simulink model "Appl_HeatAdj_CtrlModel"  (R2018b)
settings: configuration reference "CodeConfig_10_ms" (kept outside this file)
undefined symbols (not defined in the file): CAL_LEVEL3_TIMEOUT, CAL_SW_20min_TIMEOUT, D_1stLevel_36, D_2ndLevel_39, D_3rdLevel_45, D_3rdLevel_48, D_DRVHEAT_PID_D, D_DRVHEAT_PID_I, D_DRVHEAT_PID_P, D_HEAT_HEAT_DEF, D_SwsLevel_Temp, FALSE, TRUE
libraries: DareLib x111, simulink x1
(part 1 of 6)
settings Model: Creator=Administrator  LastModifiedBy=Administrator
settings ConfigSetRef: SourceLocation=Base Workspace

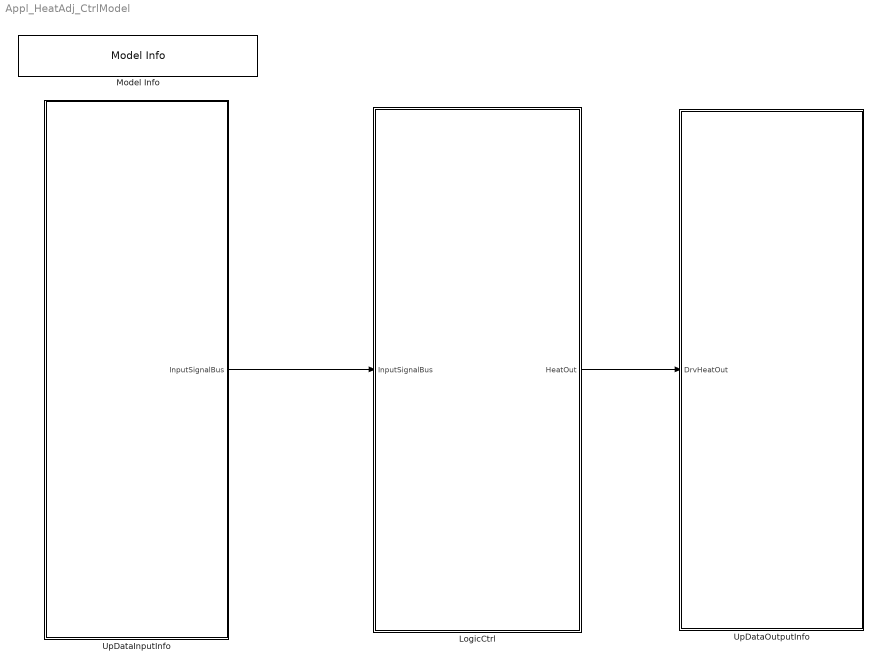
== system Appl_HeatAdj_CtrlModel ==
  LogicCtrl : Subsystem  Priority=2  TreatAsAtomicUnit=on
      settings: RTWSystemCode=Nonreusable function  RTWFcnNameOpts=Use subsystem name
  Model Info : simulink/Model-Wide Utilities/Model Info  Frame=on  DisplayStringWithTags=Version：%<ModelVersion>  HorizontalTextAlignment=Center  LeftAlignmentValue=0.5
  UpDataInputInfo : Subsystem  Priority=1  TreatAsAtomicUnit=on
      settings: RTWSystemCode=Nonreusable function  RTWFcnNameOpts=Use subsystem name
  UpDataOutputInfo : Subsystem  Priority=3  TreatAsAtomicUnit=on
      settings: RTWSystemCode=Nonreusable function  RTWFcnNameOpts=Use subsystem name
  wires:
  LogicCtrl/1(HeatOut) -> UpDataOutputInfo/1(DrvHeatOut)
  UpDataInputInfo/1(InputSignalBus) -> LogicCtrl/1(InputSignalBus)

== system Appl_HeatAdj_CtrlModel/LogicCtrl ==
  InputSignalBus : Inport
  Bus Selector : BusSelector  OutputSignals=Rte_SignalBUs.HeatAdj_D_SimuIndex_DRHeat,Rte_SignalBUs.HeatAdj_D_SimuIndex_PAHeat,Rte_SignalBUs.HeatAdj_D_SimuIndex_ThirdHeat,Rte_SignalBUs.HeatAdj_DrHeatNtcAdc,Rte_SignalBUs.HeatAdj_PaHeatNtcAdc,Rte_SignalBUs.HeatAdj_ThirdHeatNtcAdc,Rte_SignalBUs.HeatAdj_CarType,Rte_SignalBUs.HeatAdj_RemoteEnableConfig,Rte_SignalBUs.HeatAdj_TboxRemoteSts,Rte_SignalBUs.HeatAdj_RemoteMsgLostFlag,Rte_SignalBUs.HeatAdj_PlatformEngineEnableConfig,Rte_SignalBUs.HeatAdj_P20_PHEV_EngineCfg,Rte_SignalBUs.HeatAdj_ECMD_EngineStatus,Rte_SignalBUs.HeatAdj_DriverCmdFaultSts,Rte_SignalBUs.HeatAdj_DriverNTCFaultSts,Rte_SignalBUs.HeatAdj_PassengerCmdFaultSts,Rte_SignalBUs.HeatAdj_PassengerNTCFaultSts,Rte_SignalBUs.HeatAdj_ThirdCmdFaultSts,Rte_SignalBUs.HeatAdj_ThirdNTCFaultSts,Rte_SignalBUs.HeatAdj_PowerMode,Rte_SignalBUs.HeatAdj_DriverHMI_Message,Rte_SignalBUs.HeatAdj_DriverTbox_Message,Rte_SignalBUs.HeatAdj_PassengerHMI_Message,Rte_SignalBUs.HeatAdj_PassengerTbox_Message,Rte_SignalBUs.HeatAdj_ThirdHMI_Message,Rte_SignalBUs.HeatAdj_ThirdTbox_Message,Rte_SignalBUs.HeatAdj_DriverDiagCmd,Rte_SignalBUs.HeatAdj_PassengerDiagCmd,Rte_SignalBUs.HeatAdj_ThirdDiagCmd,Rte_SignalBUs.HeatAdj_TimeOutPrm,Rte_SignalBUs.HeatAdj_RunMaxTime,Rte_SignalBUs.HeatAdj_VoltMode,Rte_SignalBUs.HeatAdj_RecoverDefaultFlag,Rte_SignalBUs.HeatAdj_Driver_HMI_VentilateMsg,Rte_SignalBUs.HeatAdj_Driver_Tbox_VentilateMsg,Rte_SignalBUs.HeatAdj_Passenger_HMI_VentilateMsg,Rte_SignalBUs.HeatAdj_Passenger_Tbox_VentilateMsg,Rte_SignalBUs.HeatAdj_Third_HMI_VentilateMsg,Rte_SignalBUs.HeatAdj_Third_Tbox_VentilateMsg,Rte_SignalBUs.HeatAdj_DrHeatStopReason,Rte_SignalBUs.HeatAdj_PaHeatStopReason,Rte_SignalBUs.HeatAdj_ThirdHeatStopReason,RemoteModeFlag,EngineRunningFlag,VentValid,HeatError,Rte_SignalBUs.HeatAdj_HeatMsgLostFlag,HeatRunMaxTime,HeatMessage,VehicleRunFlag,HeatConfig,VentConfig,ComPCSatisfiedFlag,Rte_SignalBUs.HeatAdj_CanDrvHeatLvl,Rte_SignalBUs.HeatAdj_CanPasHeatLvl,Rte_SignalBUs.HeatAdj_CanThirdHeatLvl,SwHeatRunMaxTime
  LocalAdjustCtrl : Subsystem  Description=加热逻辑处理
      settings: AttributesFormatString=%<Description>
  MainVent_OutputLvlSts : BusCreator  Inputs=35
  HeatOut : Outport
  wires:
  InputSignalBus/1 -> Bus Selector/1  "InputSignalBus"
  MainVent_OutputLvlSts/1 -> HeatOut/1
  LocalAdjustCtrl/1(HeatAdj_DrHeatStopReasonOut) -> MainVent_OutputLvlSts/1
  LocalAdjustCtrl/2(HeatAdj_PaHeatStopReasonOut) -> MainVent_OutputLvlSts/2
  LocalAdjustCtrl/3(HeatAdj_ThirdHeatStopReasonOut) -> MainVent_OutputLvlSts/3
  LocalAdjustCtrl/4(HeatAdj_DrHeatTypeOut) -> MainVent_OutputLvlSts/4
  LocalAdjustCtrl/5(HeatAdj_PaHeatTypeOut) -> MainVent_OutputLvlSts/5
  LocalAdjustCtrl/6(HeatAdj_ThirdHeatTypeOut) -> MainVent_OutputLvlSts/6
  LocalAdjustCtrl/7(HeatAdj_DRHeatOut) -> MainVent_OutputLvlSts/7
  LocalAdjustCtrl/8(HeatAdj_PAHeatOut) -> MainVent_OutputLvlSts/8
  LocalAdjustCtrl/9(HeatAdj_ThirdHeatOut) -> MainVent_OutputLvlSts/9
  LocalAdjustCtrl/10(HeatAdj_DRHeatIoOut) -> MainVent_OutputLvlSts/10
  LocalAdjustCtrl/11(HeatAdj_PAHeatIoOut) -> MainVent_OutputLvlSts/11
  LocalAdjustCtrl/12(HeatAdj_ThirdHeatIoOut) -> MainVent_OutputLvlSts/12
  LocalAdjustCtrl/13(HeatAdj_DRHeatPwmOut) -> MainVent_OutputLvlSts/13
  LocalAdjustCtrl/14(HeatAdj_PAHeatPwmOut) -> MainVent_OutputLvlSts/14
  LocalAdjustCtrl/15(HeatAdj_ThirdHeatPwmOut) -> MainVent_OutputLvlSts/15
  LocalAdjustCtrl/16(HeatAdj_DrRunStateOut) -> MainVent_OutputLvlSts/16
  LocalAdjustCtrl/17(HeatAdj_PaRunStateOut) -> MainVent_OutputLvlSts/17
  LocalAdjustCtrl/18(HeatAdj_3rdRunStateOut) -> MainVent_OutputLvlSts/18
  LocalAdjustCtrl/19(EngineRunningFlagOut) -> MainVent_OutputLvlSts/19
  LocalAdjustCtrl/20(RemoteModeFlagOut) -> MainVent_OutputLvlSts/20
  LocalAdjustCtrl/21(VehicleRunFlagOut) -> MainVent_OutputLvlSts/21
  LocalAdjustCtrl/22(DiagDrHeatLevel) -> MainVent_OutputLvlSts/22
  LocalAdjustCtrl/23(DiagPaHeatLevel) -> MainVent_OutputLvlSts/23
  LocalAdjustCtrl/24(Diag3rdHeatLevel) -> MainVent_OutputLvlSts/24
  LocalAdjustCtrl/25(CANDrHeatStopReasonOut) -> MainVent_OutputLvlSts/25
  LocalAdjustCtrl/26(CAN3rdHeatStopReasonOut) -> MainVent_OutputLvlSts/26
  LocalAdjustCtrl/27(CANPaHeatStopReasonOut) -> MainVent_OutputLvlSts/27
  LocalAdjustCtrl/28(DrHeatConfigOut) -> MainVent_OutputLvlSts/28
  LocalAdjustCtrl/29(PaHeatConfigOut) -> MainVent_OutputLvlSts/29
  LocalAdjustCtrl/30(ThirdHeatConfigOut) -> MainVent_OutputLvlSts/30
  LocalAdjustCtrl/31(DrVentConfigOut) -> MainVent_OutputLvlSts/31
  LocalAdjustCtrl/32(PaVentConfigOut) -> MainVent_OutputLvlSts/32
  LocalAdjustCtrl/33(ThirdVentConfigOut) -> MainVent_OutputLvlSts/33
  LocalAdjustCtrl/34(ComPCSatisfiedFlagOut) -> MainVent_OutputLvlSts/34
  Bus Selector/1 -> LocalAdjustCtrl/1(HeatAdj_D_SimuIndex_DRHeat)  "<HeatAdj_D_SimuIndex_DRHeat>"
  Bus Selector/2 -> LocalAdjustCtrl/2(HeatAdj_D_SimuIndex_PAHeat)  "<HeatAdj_D_SimuIndex_PAHeat>"
  Bus Selector/3 -> LocalAdjustCtrl/3(HeatAdj_D_SimuIndex_ThirdHeat)  "<HeatAdj_D_SimuIndex_ThirdHeat>"
  Bus Selector/4 -> LocalAdjustCtrl/4(HeatAdj_DrHeatNtcAdc)  "<HeatAdj_DrHeatNtcAdc>"
  Bus Selector/5 -> LocalAdjustCtrl/5(HeatAdj_PaHeatNtcAdc)  "<HeatAdj_PaHeatNtcAdc>"
  Bus Selector/6 -> LocalAdjustCtrl/6(HeatAdj_ThirdHeatNtcAdc)  "<HeatAdj_ThirdHeatNtcAdc>"
  Bus Selector/7 -> LocalAdjustCtrl/7(HeatAdj_CarType)  "<HeatAdj_CarType>"
  Bus Selector/8 -> LocalAdjustCtrl/8(HeatAdj_RemoteEnableConfig)  "<HeatAdj_RemoteEnableConfig>"
  Bus Selector/9 -> LocalAdjustCtrl/9(HeatAdj_TboxRemoteSts)  "<HeatAdj_TboxRemoteSts>"
  Bus Selector/10 -> LocalAdjustCtrl/10(HeatAdj_RemoteMsgLostFlag)  "<HeatAdj_RemoteMsgLostFlag>"
  Bus Selector/11 -> LocalAdjustCtrl/11(HeatAdj_PlatformEngineEnableConfig)  "<HeatAdj_PlatformEngineEnableConfig>"
  Bus Selector/12 -> LocalAdjustCtrl/12(HeatAdj_P20_PHEV_EngineCfg)  "<HeatAdj_P20_PHEV_EngineCfg>"
  Bus Selector/13 -> LocalAdjustCtrl/13(HeatAdj_ECMD_EngineStatus)  "<HeatAdj_ECMD_EngineStatus>"
  Bus Selector/14 -> LocalAdjustCtrl/14(HeatAdj_DriverCmdFaultSts)  "<HeatAdj_DriverCmdFaultSts>"
  Bus Selector/15 -> LocalAdjustCtrl/15(HeatAdj_DriverNTCFaultSts)  "<HeatAdj_DriverNTCFaultSts>"
  Bus Selector/16 -> LocalAdjustCtrl/16(HeatAdj_PassengerCmdFaultSts)  "<HeatAdj_PassengerCmdFaultSts>"
  Bus Selector/17 -> LocalAdjustCtrl/17(HeatAdj_PassengerNTCFaultSts)  "<HeatAdj_PassengerNTCFaultSts>"
  Bus Selector/18 -> LocalAdjustCtrl/18(HeatAdj_ThirdCmdFaultSts)  "<HeatAdj_ThirdCmdFaultSts>"
  Bus Selector/19 -> LocalAdjustCtrl/19(HeatAdj_ThirdNTCFaultSts)  "<HeatAdj_ThirdNTCFaultSts>"
  Bus Selector/20 -> LocalAdjustCtrl/20(HeatAdj_PowerMode)  "<HeatAdj_PowerMode>"
  Bus Selector/21 -> LocalAdjustCtrl/21(HeatAdj_DriverHMI_Message)  "<HeatAdj_DriverHMI_Message>"
  Bus Selector/22 -> LocalAdjustCtrl/22(HeatAdj_DriverTbox_Message)  "<HeatAdj_DriverTbox_Message>"
  Bus Selector/23 -> LocalAdjustCtrl/23(HeatAdj_PassengerHMI_Message)  "<HeatAdj_PassengerHMI_Message>"
  Bus Selector/24 -> LocalAdjustCtrl/24(HeatAdj_PassengerTbox_Message)  "<HeatAdj_PassengerTbox_Message>"
  Bus Selector/25 -> LocalAdjustCtrl/25(HeatAdj_ThirdHMI_Message)  "<HeatAdj_ThirdHMI_Message>"
  Bus Selector/26 -> LocalAdjustCtrl/26(HeatAdj_ThirdTbox_Message)  "<HeatAdj_ThirdTbox_Message>"
  Bus Selector/27 -> LocalAdjustCtrl/27(HeatAdj_DriverDiagCmd)  "<HeatAdj_DriverDiagCmd>"
  Bus Selector/28 -> LocalAdjustCtrl/28(HeatAdj_PassengerDiagCmd)  "<HeatAdj_PassengerDiagCmd>"
  Bus Selector/29 -> LocalAdjustCtrl/29(HeatAdj_ThirdDiagCmd)  "<HeatAdj_ThirdDiagCmd>"
  Bus Selector/30 -> LocalAdjustCtrl/30(HeatAdj_TimeOutPrm)  "<HeatAdj_TimeOutPrm>"
  Bus Selector/31 -> LocalAdjustCtrl/31(HeatAdj_RunMaxTime)  "<HeatAdj_RunMaxTime>"
  Bus Selector/32 -> LocalAdjustCtrl/32(HeatAdj_VoltMode)  "<HeatAdj_VoltMode>"
  Bus Selector/33 -> LocalAdjustCtrl/33(HeatAdj_RecoverDefaultFlag)  "<HeatAdj_RecoverDefaultFlag>"
  Bus Selector/34 -> LocalAdjustCtrl/34(HeatAdj_Driver_HMI_VentilateMsg)  "<HeatAdj_Driver_HMI_VentilateMsg>"
  Bus Selector/35 -> LocalAdjustCtrl/35(HeatAdj_Driver_Tbox_VentilateMsg)  "<HeatAdj_Driver_Tbox_VentilateMsg>"
  Bus Selector/36 -> LocalAdjustCtrl/36(HeatAdj_Passenger_HMI_VentilateMsg)  "<HeatAdj_Passenger_HMI_VentilateMsg>"
  Bus Selector/37 -> LocalAdjustCtrl/37(HeatAdj_Passenger_Tbox_VentilateMsg)  "<HeatAdj_Passenger_Tbox_VentilateMsg>"
  Bus Selector/38 -> LocalAdjustCtrl/38(HeatAdj_Third_HMI_VentilateMsg)  "<HeatAdj_Third_HMI_VentilateMsg>"
  Bus Selector/39 -> LocalAdjustCtrl/39(HeatAdj_Third_Tbox_VentilateMsg)  "<HeatAdj_Third_Tbox_VentilateMsg>"
  Bus Selector/40 -> LocalAdjustCtrl/40(HeatAdj_DrHeatStopReason)  "<HeatAdj_DrHeatStopReason>"
  Bus Selector/41 -> LocalAdjustCtrl/41(HeatAdj_PaHeatStopReason)  "<HeatAdj_PaHeatStopReason>"
  Bus Selector/42 -> LocalAdjustCtrl/42(HeatAdj_ThirdHeatStopReason)  "<HeatAdj_ThirdHeatStopReason>"
  Bus Selector/43 -> LocalAdjustCtrl/43(RemoteModeFlag)  "<RemoteModeFlag>"
  Bus Selector/44 -> LocalAdjustCtrl/44(EngineRunningFlag)  "<EngineRunningFlag>"
  Bus Selector/45 -> LocalAdjustCtrl/45(VentValid)  "<VentValid>"
  Bus Selector/46 -> LocalAdjustCtrl/46(HeatError)  "<HeatError>"
  Bus Selector/47 -> LocalAdjustCtrl/47(HeatAdj_HeatMsgLostFlag)  "<HeatAdj_HeatMsgLostFlag>"
  Bus Selector/48 -> LocalAdjustCtrl/48(HeatRunMaxTime)  "<HeatRunMaxTime>"
  Bus Selector/49 -> LocalAdjustCtrl/49(HeatMessage)  "<HeatMessage>"
  Bus Selector/50 -> LocalAdjustCtrl/50(VehicleRunFlag)  "<VehicleRunFlag>"
  Bus Selector/51 -> LocalAdjustCtrl/51(HeatConfig)  "<HeatConfig>"
  Bus Selector/52 -> LocalAdjustCtrl/52(VentConfig)  "<VentConfig>"
  Bus Selector/53 -> LocalAdjustCtrl/53(ComPCSatisfiedFlag)  "<ComPCSatisfiedFlag>"
  Bus Selector/54 -> LocalAdjustCtrl/54(HeatAdj_CanDrvHeatLvl)  "<HeatAdj_CanDrvHeatLvl>"
  Bus Selector/55 -> LocalAdjustCtrl/55(HeatAdj_CanPasHeatLvl)  "<HeatAdj_CanPasHeatLvl>"
  Bus Selector/56 -> LocalAdjustCtrl/56(HeatAdj_CanThirdHeatLvl)  "<HeatAdj_CanThirdHeatLvl>"
  Bus Selector/57 -> LocalAdjustCtrl/57(SwHeatRunMaxTime)  "<SwHeatRunMaxTime>"
  LocalAdjustCtrl/35(Sw20minTimerOut) -> MainVent_OutputLvlSts/35  "Sw20minTimerOut"

== system Appl_HeatAdj_CtrlModel/UpDataInputInfo ==
  InputSignalProcess : Subsystem  Description=数据处理
      settings: AttributesFormatString=%<Description>  RTWSystemCode=Nonreusable function  RTWFcnNameOpts=Use subsystem name
  RTE : Subsystem  Description=接口自动生成  TreatAsAtomicUnit=on
      settings: AttributesFormatString=%<Description>  RTWSystemCode=Nonreusable function  RTWFcnNameOpts=Use subsystem name
  InputSignalBus : Outport
  wires:
  RTE/1(RTE_Signal) -> InputSignalProcess/1(Rte_SignalBUs)
  InputSignalProcess/1(InputSignalBus) -> InputSignalBus/1

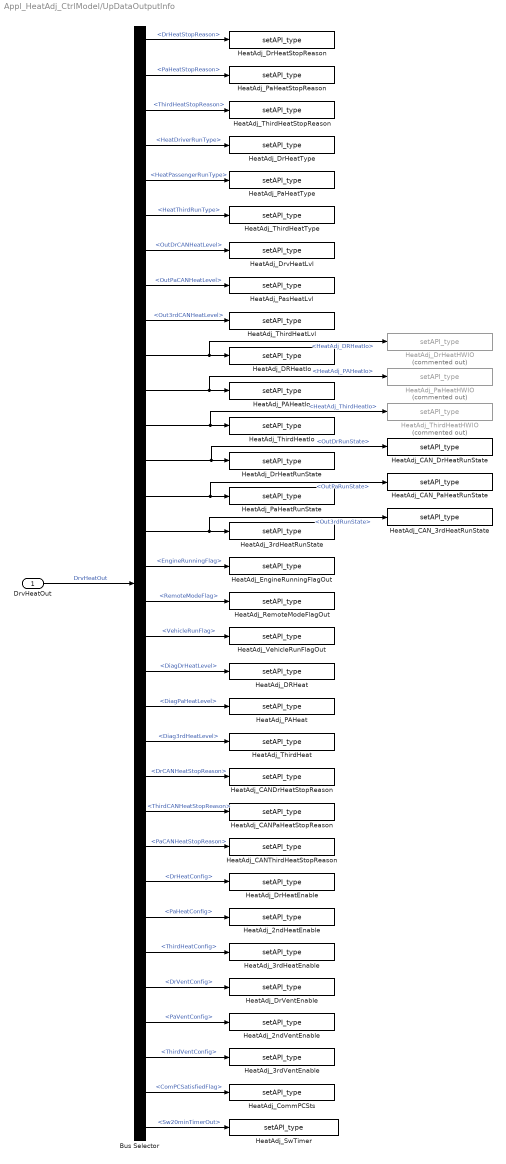
== system Appl_HeatAdj_CtrlModel/UpDataOutputInfo ==
  DrvHeatOut : Inport
  Bus Selector : BusSelector  OutputSignals=DrHeatStopReason,PaHeatStopReason,ThirdHeatStopReason,HeatDriverRunType,HeatPassengerRunType,HeatThirdRunType,OutDrCANHeatLevel,OutPaCANHeatLevel,Out3rdCANHeatLevel,HeatAdj_DRHeatIo,HeatAdj_PAHeatIo,HeatAdj_ThirdHeatIo,OutDrRunState,OutPaRunState,Out3rdRunState,EngineRunningFlag,RemoteModeFlag,VehicleRunFlag,DiagDrHeatLevel,DiagPaHeatLevel,Diag3rdHeatLevel,DrCANHeatStopReason,ThirdCANHeatStopReason,PaCANHeatStopReason,DrHeatConfig,PaHeatConfig,ThirdHeatConfig,DrVentConfig,PaVentConfig,ThirdVentConfig,ComPCSatisfiedFlag,Sw20minTimerOut
  HeatAdj_2ndHeatEnable : DareLib/Dare/setAPI_type  g_funcname=Rte_SetVfb_SecondHeatEnable  g_param=""  g_type=uint8  g_size=-1
      settings: AttributesFormatString=%<g_funcname>  SourceProductName=Dare Library
  HeatAdj_2ndVentEnable : DareLib/Dare/setAPI_type  g_funcname=Rte_SetVfb_SecondVentEnable  g_param=""  g_type=uint8  g_size=-1
      settings: AttributesFormatString=%<g_funcname>  SourceProductName=Dare Library
  HeatAdj_3rdHeatEnable : DareLib/Dare/setAPI_type  g_funcname=Rte_SetVfb_ThirdHeatEnable  g_param=""  g_type=uint8  g_size=-1
      settings: AttributesFormatString=%<g_funcname>  SourceProductName=Dare Library
  HeatAdj_3rdHeatRunState : DareLib/Dare/setAPI_type  g_funcname=Rte_SetVfb_ThirdHeatRunState  g_param=""  g_type=uint8  g_size=-1
      settings: AttributesFormatString=%<g_funcname>  SourceProductName=Dare Library
  HeatAdj_3rdVentEnable : DareLib/Dare/setAPI_type  g_funcname=Rte_SetVfb_ThirdVentEnable  g_param=""  g_type=uint8  g_size=-1
      settings: AttributesFormatString=%<g_funcname>  SourceProductName=Dare Library
  HeatAdj_CANDrHeatStopReason : DareLib/Dare/setAPI_type  g_funcname=Rte_SetVfb_CANDrHeatStopReason  g_param=""  g_type=uint8  g_enum=enHeatStopReason  g_size=-1
      settings: AttributesFormatString=%<g_funcname>  SourceProductName=Dare Library
  HeatAdj_CANPaHeatStopReason : DareLib/Dare/setAPI_type  g_funcname=Rte_SetVfb_CANPaHeatStopReason  g_param=""  g_type=uint8  g_enum=enHeatStopReason  g_size=-1
      settings: AttributesFormatString=%<g_funcname>  SourceProductName=Dare Library
  HeatAdj_CANThirdHeatStopReason : DareLib/Dare/setAPI_type  g_funcname=Rte_SetVfb_CANThirdHeatStopReason  g_param=""  g_type=uint8  g_enum=enHeatStopReason  g_size=-1
      settings: AttributesFormatString=%<g_funcname>  SourceProductName=Dare Library
  HeatAdj_CAN_3rdHeatRunState : DareLib/Dare/setAPI_type  g_funcname=Ecual_CanSetThirdHeatSts  g_param=""  g_type=uint8  g_size=-1
      settings: AttributesFormatString=%<g_funcname>  SourceProductName=Dare Library
  HeatAdj_CAN_DrHeatRunState : DareLib/Dare/setAPI_type  g_funcname=Ecual_CanSetDrvHeatSts  g_param=""  g_type=uint8  g_size=-1
      settings: AttributesFormatString=%<g_funcname>  SourceProductName=Dare Library
  HeatAdj_CAN_PaHeatRunState : DareLib/Dare/setAPI_type  g_funcname=Ecual_CanSetPasHeatSts  g_param=""  g_type=uint8  g_size=-1
      settings: AttributesFormatString=%<g_funcname>  SourceProductName=Dare Library
  HeatAdj_CommPCSts : DareLib/Dare/setAPI_type  g_funcname=Rte_SetVfb_HVCommPC  g_param=""  g_type=uint8  g_size=-1
      settings: AttributesFormatString=%<g_funcname>  SourceProductName=Dare Library
  HeatAdj_DRHeat : DareLib/Dare/setAPI_type  g_funcname=Rte_SetVfb_DrHeat  g_param=""  g_type=uint8  g_enum=enHeatLvlSts  g_size=-1
      settings: AttributesFormatString=%<g_funcname>  SourceProductName=Dare Library
  HeatAdj_DRHeatIo : DareLib/Dare/setAPI_type  g_funcname=Rte_SetVfb_DrHeatIo  g_param=""  g_type=uint8  g_enum=enHeatIoSts  g_size=-1
      settings: AttributesFormatString=%<g_funcname>  SourceProductName=Dare Library
  HeatAdj_DrHeatEnable : DareLib/Dare/setAPI_type  g_funcname=Rte_SetVfb_DrHeatEnable  g_param=""  g_type=uint8  g_size=-1
      settings: AttributesFormatString=%<g_funcname>  SourceProductName=Dare Library
  HeatAdj_DrHeatHWIO : DareLib/Dare/setAPI_type  Commented=on  g_funcname=Ecual_GpioWriteCh  g_param=""  g_type=uint8  g_enum=enHeatIoSts  g_size=-1
      settings: AttributesFormatString=%<g_funcname>  SourceProductName=Dare Library
  HeatAdj_DrHeatRunState : DareLib/Dare/setAPI_type  g_funcname=Rte_SetVfb_DrHeatRunState  g_param=""  g_type=uint8  g_size=-1
      settings: AttributesFormatString=%<g_funcname>  SourceProductName=Dare Library
  HeatAdj_DrHeatStopReason : DareLib/Dare/setAPI_type  g_funcname=Rte_SetVfb_DrHeatStopReason  g_param=""  g_type=uint8  g_enum=enHeatStopReason  g_size=-1
      settings: AttributesFormatString=%<g_funcname>  SourceProductName=Dare Library
  HeatAdj_DrHeatType : DareLib/Dare/setAPI_type  g_funcname=Rte_SetVfb_DrHeatType  g_param=""  g_type=uint8  g_enum=enHeatType  g_size=-1
      settings: AttributesFormatString=%<g_funcname>  SourceProductName=Dare Library
  HeatAdj_DrVentEnable : DareLib/Dare/setAPI_type  g_funcname=Rte_SetVfb_DrVentEnable  g_param=""  g_type=uint8  g_size=-1
      settings: AttributesFormatString=%<g_funcname>  SourceProductName=Dare Library
  HeatAdj_DrvHeatLvl : DareLib/Dare/setAPI_type  g_funcname=CanTx_0x3B2_DSM_St_DriSeatHeatGear  g_param=""  g_type=uint8  g_enum=enHeatLvlSts  g_size=-1
      settings: AttributesFormatString=%<g_funcname>  SourceProductName=Dare Library
  HeatAdj_EngineRunningFlagOut : DareLib/Dare/setAPI_type  g_funcname=Rte_SetVfb_EngineRunFlag  g_param=""  g_type=uint8  g_size=-1
      settings: AttributesFormatString=%<g_funcname>  SourceProductName=Dare Library
  HeatAdj_PAHeat : DareLib/Dare/setAPI_type  g_funcname=Rte_SetVfb_PaHeat  g_param=""  g_type=uint8  g_enum=enHeatLvlSts  g_size=-1
      settings: AttributesFormatString=%<g_funcname>  SourceProductName=Dare Library
  HeatAdj_PAHeatIo : DareLib/Dare/setAPI_type  g_funcname=Rte_SetVfb_PaHeatIo  g_param=""  g_type=uint8  g_enum=enHeatIoSts  g_size=-1
      settings: AttributesFormatString=%<g_funcname>  SourceProductName=Dare Library
  HeatAdj_PaHeatHWIO : DareLib/Dare/setAPI_type  Commented=on  g_funcname=Ecual_GpioWriteCh  g_param=""  g_type=uint8  g_enum=enHeatIoSts  g_size=-1
      settings: AttributesFormatString=%<g_funcname>  SourceProductName=Dare Library
  HeatAdj_PaHeatRunState : DareLib/Dare/setAPI_type  g_funcname=Rte_SetVfb_PaHeatRunState  g_param=""  g_type=uint8  g_size=-1
      settings: AttributesFormatString=%<g_funcname>  SourceProductName=Dare Library
  HeatAdj_PaHeatStopReason : DareLib/Dare/setAPI_type  g_funcname=Rte_SetVfb_PaHeatStopReason  g_param=""  g_type=uint8  g_enum=enHeatStopReason  g_size=-1
      settings: AttributesFormatString=%<g_funcname>  SourceProductName=Dare Library
  HeatAdj_PaHeatType : DareLib/Dare/setAPI_type  g_funcname=Rte_SetVfb_PaHeatType  g_param=""  g_type=uint8  g_enum=enHeatType  g_size=-1
      settings: AttributesFormatString=%<g_funcname>  SourceProductName=Dare Library
  HeatAdj_PasHeatLvl : DareLib/Dare/setAPI_type  g_funcname=CanTx_0x3B2_DSM_St_PasSeatHeatGear  g_param=""  g_type=uint8  g_enum=enHeatLvlSts  g_size=-1
      settings: AttributesFormatString=%<g_funcname>  SourceProductName=Dare Library
  HeatAdj_RemoteModeFlagOut : DareLib/Dare/setAPI_type  g_funcname=Rte_SetVfb_RemoteModeFlag  g_param=""  g_type=uint8  g_size=-1
      settings: AttributesFormatString=%<g_funcname>  SourceProductName=Dare Library
  HeatAdj_SwTimer : DareLib/Dare/setAPI_type  g_funcname=DiagSetSwHeatTimer  g_param=""  g_type=uint32  g_size=-1
      settings: AttributesFormatString=%<g_funcname>  SourceProductName=Dare Library
  HeatAdj_ThirdHeat : DareLib/Dare/setAPI_type  g_funcname=Rte_SetVfb_ThirdHeat  g_param=""  g_type=uint8  g_enum=enHeatLvlSts  g_size=-1
      settings: AttributesFormatString=%<g_funcname>  SourceProductName=Dare Library
  HeatAdj_ThirdHeatHWIO : DareLib/Dare/setAPI_type  Commented=on  g_funcname=Ecual_GpioWriteCh  g_param=""  g_type=uint8  g_enum=enHeatIoSts  g_size=-1
      settings: AttributesFormatString=%<g_funcname>  SourceProductName=Dare Library
  HeatAdj_ThirdHeatIo : DareLib/Dare/setAPI_type  g_funcname=Rte_SetVfb_ThirdHeatIo  g_param=""  g_type=uint8  g_enum=enHeatIoSts  g_size=-1
      settings: AttributesFormatString=%<g_funcname>  SourceProductName=Dare Library
  HeatAdj_ThirdHeatLvl : DareLib/Dare/setAPI_type  g_funcname=Ecual_CanSetThirdHeatLvl  g_param=""  g_type=uint8  g_enum=enHeatLvlSts  g_size=-1
      settings: AttributesFormatString=%<g_funcname>  SourceProductName=Dare Library
  HeatAdj_ThirdHeatStopReason : DareLib/Dare/setAPI_type  g_funcname=Rte_SetVfb_ThirdHeatStopReason  g_param=""  g_type=uint8  g_enum=enHeatStopReason  g_size=-1
      settings: AttributesFormatString=%<g_funcname>  SourceProductName=Dare Library
  HeatAdj_ThirdHeatType : DareLib/Dare/setAPI_type  g_funcname=Rte_SetVfb_ThirdHeatType  g_param=""  g_type=uint8  g_enum=enHeatType  g_size=-1
      settings: AttributesFormatString=%<g_funcname>  SourceProductName=Dare Library
  HeatAdj_VehicleRunFlagOut : DareLib/Dare/setAPI_type  g_funcname=Rte_SetVfb_VehicleRunFlag  g_param=""  g_type=uint8  g_size=-1
      settings: AttributesFormatString=%<g_funcname>  SourceProductName=Dare Library
  wires:
  DrvHeatOut/1 -> Bus Selector/1  "DrvHeatOut"
  Bus Selector/4 -> HeatAdj_DrHeatType/1  "<HeatDriverRunType>"
  Bus Selector/5 -> HeatAdj_PaHeatType/1  "<HeatPassengerRunType>"
  Bus Selector/6 -> HeatAdj_ThirdHeatType/1  "<HeatThirdRunType>"
  Bus Selector/3 -> HeatAdj_ThirdHeatStopReason/1  "<ThirdHeatStopReason>"
  Bus Selector/2 -> HeatAdj_PaHeatStopReason/1  "<PaHeatStopReason>"
  Bus Selector/1 -> HeatAdj_DrHeatStopReason/1  "<DrHeatStopReason>"
  Bus Selector/7 -> HeatAdj_DrvHeatLvl/1  "<OutDrCANHeatLevel>"
  Bus Selector/8 -> HeatAdj_PasHeatLvl/1  "<OutPaCANHeatLevel>"
  Bus Selector/9 -> HeatAdj_ThirdHeatLvl/1  "<Out3rdCANHeatLevel>"
  Bus Selector/10 -> HeatAdj_DRHeatIo/1, HeatAdj_DrHeatHWIO/1  "<HeatAdj_DRHeatIo>"
  Bus Selector/11 -> HeatAdj_PAHeatIo/1, HeatAdj_PaHeatHWIO/1  "<HeatAdj_PAHeatIo>"
  Bus Selector/12 -> HeatAdj_ThirdHeatHWIO/1, HeatAdj_ThirdHeatIo/1  "<HeatAdj_ThirdHeatIo>"
  Bus Selector/17 -> HeatAdj_RemoteModeFlagOut/1  "<RemoteModeFlag>"
  Bus Selector/16 -> HeatAdj_EngineRunningFlagOut/1  "<EngineRunningFlag>"
  Bus Selector/13 -> HeatAdj_CAN_DrHeatRunState/1, HeatAdj_DrHeatRunState/1  "<OutDrRunState>"
  Bus Selector/18 -> HeatAdj_VehicleRunFlagOut/1  "<VehicleRunFlag>"
  Bus Selector/19 -> HeatAdj_DRHeat/1  "<DiagDrHeatLevel>"
  Bus Selector/20 -> HeatAdj_PAHeat/1  "<DiagPaHeatLevel>"
  Bus Selector/21 -> HeatAdj_ThirdHeat/1  "<Diag3rdHeatLevel>"
  Bus Selector/14 -> HeatAdj_CAN_PaHeatRunState/1, HeatAdj_PaHeatRunState/1  "<OutPaRunState>"
  Bus Selector/15 -> HeatAdj_CAN_3rdHeatRunState/1, HeatAdj_3rdHeatRunState/1  "<Out3rdRunState>"
  Bus Selector/22 -> HeatAdj_CANDrHeatStopReason/1  "<DrCANHeatStopReason>"
  Bus Selector/23 -> HeatAdj_CANPaHeatStopReason/1  "<ThirdCANHeatStopReason>"
  Bus Selector/24 -> HeatAdj_CANThirdHeatStopReason/1  "<PaCANHeatStopReason>"
  Bus Selector/25 -> HeatAdj_DrHeatEnable/1  "<DrHeatConfig>"
  Bus Selector/26 -> HeatAdj_2ndHeatEnable/1  "<PaHeatConfig>"
  Bus Selector/27 -> HeatAdj_3rdHeatEnable/1  "<ThirdHeatConfig>"
  Bus Selector/28 -> HeatAdj_DrVentEnable/1  "<DrVentConfig>"
  Bus Selector/29 -> HeatAdj_2ndVentEnable/1  "<PaVentConfig>"
  Bus Selector/30 -> HeatAdj_3rdVentEnable/1  "<ThirdVentConfig>"
  Bus Selector/31 -> HeatAdj_CommPCSts/1  "<ComPCSatisfiedFlag>"
  Bus Selector/32 -> HeatAdj_SwTimer/1  "<Sw20minTimerOut>"

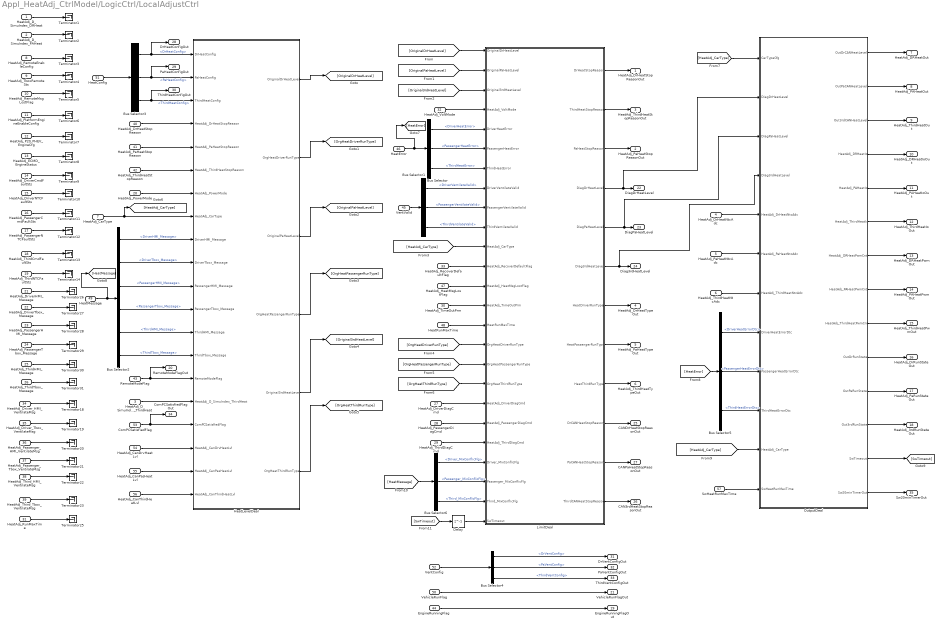
== system Appl_HeatAdj_CtrlModel/LogicCtrl/LocalAdjustCtrl ==
  HeatAdj_D_SimuIndex_DRHeat : Inport
  HeatAdj_D_SimuIndex_PAHeat : Inport  Port=2
  HeatAdj_D_SimuIndex_ThirdHeat : Inport  Port=3
  HeatAdj_DrHeatNtcAdc : Inport  Port=4
  HeatAdj_PaHeatNtcAdc : Inport  Port=5
  HeatAdj_ThirdHeatNtcAdc : Inport  Port=6
  HeatAdj_CarType : Inport  Port=7
  HeatAdj_RemoteEnableConfig : Inport  Port=8
  HeatAdj_TboxRemoteSts : Inport  Port=9
  HeatAdj_RemoteMsgLostFlag : Inport  Port=10
  HeatAdj_PlatformEngineEnableConfig : Inport  Port=11
  HeatAdj_P20_PHEV_EngineCfg : Inport  Port=12
  HeatAdj_ECMD_EngineStatus : Inport  Port=13
  HeatAdj_DriverCmdFaultSts : Inport  Port=14
  HeatAdj_DriverNTCFaultSts : Inport  Port=15
  HeatAdj_PassengerCmdFaultSts : Inport  Port=16
  HeatAdj_PassengerNTCFaultSts : Inport  Port=17
  HeatAdj_ThirdCmdFaultSts : Inport  Port=18
  HeatAdj_ThirdNTCFaultSts : Inport  Port=19
  HeatAdj_PowerMode : Inport  Port=20
  HeatAdj_DriverHMI_Message : Inport  Port=21
  HeatAdj_DriverTbox_Message : Inport  Port=22
  HeatAdj_PassengerHMI_Message : Inport  Port=23
  HeatAdj_PassengerTbox_Message : Inport  Port=24
  HeatAdj_ThirdHMI_Message : Inport  Port=25
  HeatAdj_ThirdTbox_Message : Inport  Port=26
  HeatAdj_DriverDiagCmd : Inport  Port=27
  HeatAdj_PassengerDiagCmd : Inport  Port=28
  HeatAdj_ThirdDiagCmd : Inport  Port=29
  HeatAdj_TimeOutPrm : Inport  Port=30
  HeatAdj_RunMaxTime : Inport  Port=31
  HeatAdj_VoltMode : Inport  Port=32
  HeatAdj_RecoverDefaultFlag : Inport  Port=33
  HeatAdj_Driver_HMI_VentilateMsg : Inport  Port=34
  HeatAdj_Driver_Tbox_VentilateMsg : Inport  Port=35
  HeatAdj_Passenger_HMI_VentilateMsg : Inport  Port=36
  HeatAdj_Passenger_Tbox_VentilateMsg : Inport  Port=37
  HeatAdj_Third_HMI_VentilateMsg : Inport  Port=38
  HeatAdj_Third_Tbox_VentilateMsg : Inport  Port=39
  HeatAdj_DrHeatStopReason : Inport  Port=40
  HeatAdj_PaHeatStopReason : Inport  Port=41
  HeatAdj_ThirdHeatStopReason : Inport  Port=42
  RemoteModeFlag : Inport  Port=43
  EngineRunningFlag : Inport  Port=44
  VentValid : Inport  Port=45
  HeatError : Inport  Port=46
  HeatAdj_HeatMsgLostFlag : Inport  Port=47
  HeatRunMaxTime : Inport  Port=48
  HeatMessage : Inport  Port=49
  VehicleRunFlag : Inport  Port=50
  HeatConfig : Inport  Port=51
  VentConfig : Inport  Port=52
  ComPCSatisfiedFlag : Inport  Port=53
  HeatAdj_CanDrvHeatLvl : Inport  Port=54
  HeatAdj_CanPasHeatLvl : Inport  Port=55
  HeatAdj_CanThirdHeatLvl : Inport  Port=56
  SwHeatRunMaxTime : Inport  Port=57
  Bus Selector : BusSelector  OutputSignals=DriverHeatError,PassengerHeatError,ThirdHeatError
  Bus Selector1 : BusSelector  OutputSignals=DriverVentilateValid,PassengerVentilateValid,ThirdVentilateValid
  Bus Selector2 : BusSelector  OutputSignals=DriverHMI_Message,DriverTbox_Message,PassengerHMI_Message,PassengerTbox_Message,ThirdHMI_Message,ThirdTbox_Message
  Bus Selector3 : BusSelector  OutputSignals=DrHeatConfig,PaHeatConfig,ThirdHeatConfig
  Bus Selector4 : BusSelector  OutputSignals=DrVentConfig,PaVentConfig,ThirdVentConfig
  Bus Selector5 : BusSelector  OutputSignals=DriverHeatErrorDtc,PassengerHeatErrorDtc,ThirdHeatErrorDtc
  Bus Selector6 : BusSelector  OutputSignals=Driver_MixConflicFlg,Passenger_MixConflicFlg,Third_MixConflicFlg
  Delay : Delay  DelayLength=1  InitialCondition=0
  HeatLevelDeal : Stateflow chart  TreatAsAtomicUnit=on
  LimitDeal : Stateflow chart  TreatAsAtomicUnit=on
  OutputDeal : Stateflow chart  TreatAsAtomicUnit=on
  Terminator{1..14,18..23,25..31} (27 alike) : Terminator
  HeatAdj_DrHeatStopReasonOut : Outport
  HeatAdj_PaHeatStopReasonOut : Outport  Port=2
  HeatAdj_ThirdHeatStopReasonOut : Outport  Port=3
  HeatAdj_DrHeatTypeOut : Outport  Port=4
  HeatAdj_PaHeatTypeOut : Outport  Port=5
  HeatAdj_ThirdHeatTypeOut : Outport  Port=6
  HeatAdj_DRHeatOut : Outport  Port=7
  HeatAdj_PAHeatOut : Outport  Port=8
  HeatAdj_ThirdHeatOut : Outport  Port=9
  HeatAdj_DRHeatIoOut : Outport  Port=10
  HeatAdj_PAHeatIoOut : Outport  Port=11
  HeatAdj_ThirdHeatIoOut : Outport  Port=12
  HeatAdj_DRHeatPwmOut : Outport  Port=13
  HeatAdj_PAHeatPwmOut : Outport  Port=14
  HeatAdj_ThirdHeatPwmOut : Outport  Port=15
  HeatAdj_DrRunStateOut : Outport  Port=16
  HeatAdj_PaRunStateOut : Outport  Port=17
  HeatAdj_3rdRunStateOut : Outport  Port=18
  EngineRunningFlagOut : Outport  Port=19
  RemoteModeFlagOut : Outport  Port=20
  VehicleRunFlagOut : Outport  Port=21
  DiagDrHeatLevel : Outport  Port=22
  DiagPaHeatLevel : Outport  Port=23
  Diag3rdHeatLevel : Outport  Port=24
  CANDrHeatStopReasonOut : Outport  Port=25
  CAN3rdHeatStopReasonOut : Outport  Port=26
  CANPaHeatStopReasonOut : Outport  Port=27
  DrHeatConfigOut : Outport  Port=28
  PaHeatConfigOut : Outport  Port=29
  ThirdHeatConfigOut : Outport  Port=30
  DrVentConfigOut : Outport  Port=31
  PaVentConfigOut : Outport  Port=32
  ThirdVentConfigOut : Outport  Port=33
  ComPCSatisfiedFlagOut : Outport  Port=34
  Sw20minTimerOut : Outport  Port=35
  wires:
  HeatAdj_CarType/1 -> [HeatAdj_CarType], HeatLevelDeal/8(HeatAdj_CarType)
  HeatAdj_PowerMode/1 -> HeatLevelDeal/7(HeatAdj_PowerMode)
  HeatAdj_ThirdHeatStopReason/1 -> HeatLevelDeal/6(HeatAdj_ThirdHeatStopReason)
  HeatAdj_PaHeatStopReason/1 -> HeatLevelDeal/5(HeatAdj_PaHeatStopReason)
  HeatAdj_DrHeatStopReason/1 -> HeatLevelDeal/4(HeatAdj_DrHeatStopReason)
  EngineRunningFlag/1 -> EngineRunningFlagOut/1
  RemoteModeFlag/1 -> RemoteModeFlagOut/1, HeatLevelDeal/15(RemoteModeFlag)
  HeatLevelDeal/1(OriginalDrHeatLevel) -> [OriginalDrHeatLevel]
  HeatLevelDeal/2(OrgHeatDriverRunType) -> [OrgHeatDriverRunType]
  HeatLevelDeal/3(OriginalPaHeatLevel) -> [OriginalPaHeatLevel]
  HeatLevelDeal/4(OrgHeatPassengerRunType) -> [OrgHeatPassengerRunType]
  HeatLevelDeal/5(Original3rdHeatLevel) -> [Original3rdHeatLevel]
  HeatLevelDeal/6(OrgHeatThirdRunType) -> [OrgHeatThirdRunType]
  [OriginalDrHeatLevel] -> LimitDeal/1(OriginalDrHeatLevel)
  [OriginalPaHeatLevel] -> LimitDeal/2(OriginalPaHeatLevel)
  [Original3rdHeatLevel] -> LimitDeal/3(Original3rdHeatLevel)
  HeatAdj_VoltMode/1 -> LimitDeal/4(HeatAdj_VoltMode)
  HeatError/1 -> [HeatError], Bus Selector/1
  Bus Selector/2 -> LimitDeal/6(PassengerHeatError)  "<PassengerHeatError>"
  Bus Selector/1 -> LimitDeal/5(DriverHeatError)  "<DriverHeatError>"
  Bus Selector/3 -> LimitDeal/7(ThirdHeatError)  "<ThirdHeatError>"
  VentValid/1 -> Bus Selector1/1
  Bus Selector1/2 -> LimitDeal/9(PassengerVentilateValid)  "<PassengerVentilateValid>"
  Bus Selector1/1 -> LimitDeal/8(DriverVentilateValid)  "<DriverVentilateValid>"
  Bus Selector1/3 -> LimitDeal/10(ThirdVentilateValid)  "<ThirdVentilateValid>"
  [HeatAdj_CarType] -> LimitDeal/11(HeatAdj_CarType)
  HeatAdj_RecoverDefaultFlag/1 -> LimitDeal/12(HeatAdj_RecoverDefaultFlag)
  HeatAdj_TimeOutPrm/1 -> LimitDeal/14(HeatAdj_TimeOutPrm)
  [OrgHeatDriverRunType] -> LimitDeal/16(OrgHeatDriverRunType)
  [OrgHeatPassengerRunType] -> LimitDeal/17(OrgHeatPassengerRunType)
  [OrgHeatThirdRunType] -> LimitDeal/18(OrgHeatThirdRunType)
  HeatAdj_DriverDiagCmd/1 -> LimitDeal/19(HeatAdj_DriverDiagCmd)
  HeatAdj_PassengerDiagCmd/1 -> LimitDeal/20(HeatAdj_PassengerDiagCmd)
  HeatAdj_ThirdDiagCmd/1 -> LimitDeal/21(HeatAdj_ThirdDiagCmd)
  LimitDeal/1(DrHeatStopReason) -> HeatAdj_DrHeatStopReasonOut/1
  LimitDeal/3(PaHeatStopReason) -> HeatAdj_PaHeatStopReasonOut/1
  LimitDeal/2(ThirdHeatStopReason) -> HeatAdj_ThirdHeatStopReasonOut/1
  [HeatAdj_CarType] -> OutputDeal/1(CarTypeCfg)
  LimitDeal/4(DiagDrHeatLevel) -> DiagDrHeatLevel/1, OutputDeal/2(DiagDrHeatLevel)
  LimitDeal/5(DiagPaHeatLevel) -> DiagPaHeatLevel/1, OutputDeal/3(DiagPaHeatLevel)
  LimitDeal/6(Diag3rdHeatLevel) -> OutputDeal/4(Diag3rdHeatLevel), Diag3rdHeatLevel/1
  LimitDeal/7(HeatDriverRunType) -> HeatAdj_DrHeatTypeOut/1
  LimitDeal/8(HeatPassengerRunType) -> HeatAdj_PaHeatTypeOut/1
  LimitDeal/9(HeatThirdRunType) -> HeatAdj_ThirdHeatTypeOut/1
  OutputDeal/1(OutDrCANHeatLevel) -> HeatAdj_DRHeatOut/1
  OutputDeal/2(OutPaCANHeatLevel) -> HeatAdj_PAHeatOut/1
  OutputDeal/3(Out3rdCANHeatLevel) -> HeatAdj_ThirdHeatOut/1
  OutputDeal/4(HeatAdj_DRHeatIo) -> HeatAdj_DRHeatIoOut/1
  OutputDeal/5(HeatAdj_PAHeatIo) -> HeatAdj_PAHeatIoOut/1
  OutputDeal/6(HeatAdj_ThirdHeatIo) -> HeatAdj_ThirdHeatIoOut/1
  OutputDeal/8(HeatAdj_PAHeatPwmCnt) -> HeatAdj_PAHeatPwmOut/1
  OutputDeal/9(HeatAdj_ThirdHeatPwmCnt) -> HeatAdj_ThirdHeatPwmOut/1
  OutputDeal/7(HeatAdj_DRHeatPwmCnt) -> HeatAdj_DRHeatPwmOut/1
  HeatAdj_D_SimuIndex_DRHeat/1 -> Terminator1/1
  HeatAdj_D_SimuIndex_PAHeat/1 -> Terminator2/1
  HeatAdj_D_SimuIndex_ThirdHeat/1 -> HeatLevelDeal/16(HeatAdj_D_SimuIndex_ThirdHeat)
  HeatAdj_RemoteEnableConfig/1 -> Terminator3/1
  HeatAdj_TboxRemoteSts/1 -> Terminator4/1
  HeatAdj_RemoteMsgLostFlag/1 -> Terminator5/1
  HeatAdj_PlatformEngineEnableConfig/1 -> Terminator6/1
  HeatAdj_P20_PHEV_EngineCfg/1 -> Terminator7/1
  HeatAdj_ECMD_EngineStatus/1 -> Terminator8/1
  HeatAdj_DriverCmdFaultSts/1 -> Terminator9/1
  HeatAdj_DriverNTCFaultSts/1 -> Terminator10/1
  HeatAdj_PassengerCmdFaultSts/1 -> Terminator11/1
  HeatAdj_PassengerNTCFaultSts/1 -> Terminator12/1
  HeatAdj_ThirdCmdFaultSts/1 -> Terminator13/1
  HeatAdj_ThirdNTCFaultSts/1 -> Terminator14/1
  HeatAdj_Driver_HMI_VentilateMsg/1 -> Terminator18/1
  HeatAdj_Driver_Tbox_VentilateMsg/1 -> Terminator19/1
  HeatAdj_Passenger_HMI_VentilateMsg/1 -> Terminator20/1
  HeatAdj_Passenger_Tbox_VentilateMsg/1 -> Terminator21/1
  HeatAdj_Third_HMI_VentilateMsg/1 -> Terminator22/1
  HeatAdj_Third_Tbox_VentilateMsg/1 -> Terminator23/1
  HeatAdj_HeatMsgLostFlag/1 -> LimitDeal/13(HeatAdj_HeatMsgLostFlag)
  OutputDeal/10(OutDrRunState) -> HeatAdj_DrRunStateOut/1
  OutputDeal/11(OutPaRunState) -> HeatAdj_PaRunStateOut/1
  OutputDeal/12(Out3rdRunState) -> HeatAdj_3rdRunStateOut/1
  HeatRunMaxTime/1 -> LimitDeal/15(HeatRunMaxTime)
  HeatAdj_RunMaxTime/1 -> Terminator25/1
  HeatMessage/1 -> [HeatMessage], Bus Selector2/1
  Bus Selector2/4 -> HeatLevelDeal/12(PassengerTbox_Message)  "<PassengerTbox_Message>"
  Bus Selector2/3 -> HeatLevelDeal/11(PassengerHMI_Message)  "<PassengerHMI_Message>"
  Bus Selector2/5 -> HeatLevelDeal/13(ThirdHMI_Message)  "<ThirdHMI_Message>"
  Bus Selector2/2 -> HeatLevelDeal/10(DriverTbox_Message)  "<DriverTbox_Message>"
  Bus Selector2/6 -> HeatLevelDeal/14(ThirdTbox_Message)  "<ThirdTbox_Message>"
  Bus Selector2/1 -> HeatLevelDeal/9(DriverHMI_Message)  "<DriverHMI_Message>"
  HeatAdj_ThirdHMI_Message/1 -> Terminator30/1
  HeatAdj_PassengerTbox_Message/1 -> Terminator29/1
  HeatAdj_PassengerHMI_Message/1 -> Terminator28/1
  HeatAdj_DriverTbox_Message/1 -> Terminator27/1
  HeatAdj_DriverHMI_Message/1 -> Terminator26/1
  HeatAdj_ThirdTbox_Message/1 -> Terminator31/1
  VehicleRunFlag/1 -> VehicleRunFlagOut/1
  LimitDeal/12(ThirdCANHeatStopReason) -> CAN3rdHeatStopReasonOut/1
  LimitDeal/11(PaCANHeatStopReason) -> CANPaHeatStopReasonOut/1
  LimitDeal/10(DrCANHeatStopReason) -> CANDrHeatStopReasonOut/1
  HeatConfig/1 -> Bus Selector3/1
  VentConfig/1 -> Bus Selector4/1
  Bus Selector4/1 -> DrVentConfigOut/1  "<DrVentConfig>"
  Bus Selector4/2 -> PaVentConfigOut/1  "<PaVentConfig>"
  Bus Selector4/3 -> ThirdVentConfigOut/1  "<ThirdVentConfig>"
  Bus Selector3/1 -> DrHeatConfigOut/1, HeatLevelDeal/1(DrHeatConfig)  "<DrHeatConfig>"
  Bus Selector3/2 -> PaHeatConfigOut/1, HeatLevelDeal/2(PaHeatConfig)  "<PaHeatConfig>"
  Bus Selector3/3 -> ThirdHeatConfigOut/1, HeatLevelDeal/3(ThirdHeatConfig)  "<ThirdHeatConfig>"
  ComPCSatisfiedFlag/1 -> HeatLevelDeal/17(ComPCSatisfiedFlag), ComPCSatisfiedFlagOut/1
  HeatAdj_CanDrvHeatLvl/1 -> HeatLevelDeal/18(HeatAdj_CanDrvHeatLvl)
  HeatAdj_CanPasHeatLvl/1 -> HeatLevelDeal/19(HeatAdj_CanPasHeatLvl)
  HeatAdj_CanThirdHeatLvl/1 -> HeatLevelDeal/20(HeatAdj_CanThirdHeatLvl)
  [HeatError] -> Bus Selector5/1
  HeatAdj_DrHeatNtcAdc/1 -> OutputDeal/5(HeatAdj_DrHeatNtcAdc)
  HeatAdj_PaHeatNtcAdc/1 -> OutputDeal/6(HeatAdj_PaHeatNtcAdc)
  HeatAdj_ThirdHeatNtcAdc/1 -> OutputDeal/7(HeatAdj_ThirdHeatNtcAdc)
  Bus Selector5/2 -> OutputDeal/9(PassengerHeatErrorDtc)  "<PassengerHeatErrorDtc>"
  Bus Selector5/1 -> OutputDeal/8(DriverHeatErrorDtc)  "<DriverHeatErrorDtc>"
  Bus Selector5/3 -> OutputDeal/10(ThirdHeatErrorDtc)  "<ThirdHeatErrorDtc>"
  [HeatAdj_CarType] -> OutputDeal/11(HeatAdj_CarType)
  [HeatMessage] -> Bus Selector6/1
  Bus Selector6/1 -> LimitDeal/22(Driver_MixConflicFlg)  "<Driver_MixConflicFlg>"
  Bus Selector6/2 -> LimitDeal/23(Passenger_MixConflicFlg)  "<Passenger_MixConflicFlg>"
  Bus Selector6/3 -> LimitDeal/24(Third_MixConflicFlg)  "<Third_MixConflicFlg>"
  OutputDeal/13(SwTimeout) -> [SwTimeout]
  [SwTimeout] -> Delay/1
  Delay/1 -> LimitDeal/25(SwTimeout)
  SwHeatRunMaxTime/1 -> OutputDeal/12(SwHeatRunMaxTime)
  OutputDeal/14(Sw20minTimerOut) -> Sw20minTimerOut/1

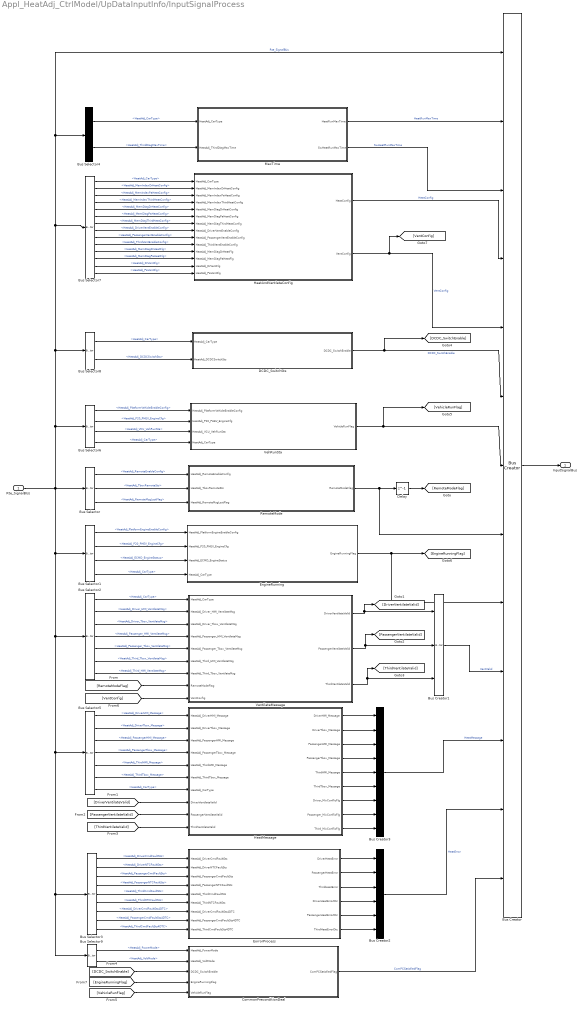
== system Appl_HeatAdj_CtrlModel/UpDataInputInfo/InputSignalProcess ==
  Rte_SignalBUs : Inport
  Bus Creator : BusCreator  Inputs=13
  Bus Creator1 : BusCreator  Inputs=3
  Bus Creator2 : BusCreator  Inputs=6
  Bus Creator3 : BusCreator  Inputs=9
  Bus Selector : BusSelector  OutputSignals=HeatAdj_RemoteEnableConfig,HeatAdj_TboxRemoteSts,HeatAdj_RemoteMsgLostFlag
  Bus Selector1 : BusSelector  OutputSignals=HeatAdj_PlatformEngineEnableConfig,HeatAdj_P20_PHEV_EngineCfg,HeatAdj_ECMD_EngineStatus,HeatAdj_CarType
  Bus Selector2 : BusSelector  OutputSignals=HeatAdj_CarType,HeatAdj_Driver_HMI_VentilateMsg,HeatAdj_Driver_Tbox_VentilateMsg,HeatAdj_Passenger_HMI_VentilateMsg,HeatAdj_Passenger_Tbox_VentilateMsg,HeatAdj_Third_Tbox_VentilateMsg,HeatAdj_Third_HMI_VentilateMsg
  Bus Selector3 : BusSelector  OutputSignals=HeatAdj_DriverCmdFaultSts,HeatAdj_DriverNTCFaultSts,HeatAdj_PassengerCmdFaultSts,HeatAdj_PassengerNTCFaultSts,HeatAdj_ThirdCmdFaultSts,HeatAdj_ThirdNTCFaultSts,HeatAdj_DriverCmdFaultSts4DTC,HeatAdj_PassengerCmdFaultSts4DTC,HeatAdj_ThirdCmdFaultSts4DTC
  Bus Selector4 : BusSelector  OutputSignals=HeatAdj_CarType,HeatAdj_ThirdDiagMaxTime
  Bus Selector5 : BusSelector  OutputSignals=HeatAdj_DriverHMI_Message,HeatAdj_DriverTbox_Message,HeatAdj_PassengerHMI_Message,HeatAdj_PassengerTbox_Message,HeatAdj_ThirdHMI_Message,HeatAdj_ThirdTbox_Message,HeatAdj_CarType
  Bus Selector6 : BusSelector  OutputSignals=HeatAdj_PlatformVehicleEnableConfig,HeatAdj_P20_PHEV_EngineCfg,HeatAdj_VCU_VehRunSta,HeatAdj_CarType
  Bus Selector7 : BusSelector  OutputSignals=HeatAdj_CarType,HeatAdj_MemIndexDrHeatConfig,HeatAdj_MemIndexPaHeatConfig,HeatAdj_MemIndexThirdHeatConfig,HeatAdj_MemDiagDrHeatConfig,HeatAdj_MemDiagPaHeatConfig,HeatAdj_MemDiagThirdHeatConfig,HeatAdj_DriverVentEnableConfig,HeatAdj_PassengerVentEnableConfig,HeatAdj_ThirdVentEnableConfig,HeatAdj_MemDiagDrHeatFlg,HeatAdj_MemDiagPaHeatFlg,HeatAdj_DrVentFlg,HeatAdj_PaVentFlg
  Bus Selector8 : BusSelector  OutputSignals=HeatAdj_CarType,HeatAdj_DCDCSwitchSts
  Bus Selector9 : BusSelector  OutputSignals=HeatAdj_PowerMode,HeatAdj_VoltMode
  CommonPreconditionDeal : Subsystem  Description=通用前置条件处理
      settings: AttributesFormatString=%<Description>
      mask Display: image('加热通用前置条件.png');
  DCDC_SwitchSts : Subsystem  Description=DCDC节点开关状态（有关实车电压）
      settings: AttributesFormatString=%<Description>
      mask Display: image('DCDC开关状态.png');
  Delay : Delay  DelayLength=1  InitialCondition=0
  EngineRunning : Subsystem  Description=发动机运行
      settings: AttributesFormatString=%<Description>
      mask Display: image('发动机运行.png');
  EorrorProcess : Subsystem  Description=故障处理
      settings: AttributesFormatString=%<Description>
      mask Display: image('故障处理.png');
  HeatAndVentlateConfig : Subsystem  Description=通风加热配置
      settings: AttributesFormatString=%<Description>
      mask Display: image('通风加热配置.png');
  HeatMessage : Subsystem  Description=加热报文处理
      settings: AttributesFormatString=%<Description>
      mask Display: image('加热报文处理.png');
  MaxTime : Subsystem  Description=最大运行时间
      settings: AttributesFormatString=%<Description>
      mask Display: image('最大运行时间.png');
  RemoteMode : Subsystem  Description=远程模式
      settings: AttributesFormatString=%<Description>
      mask Display: image('远程模式.png');
  VehRunSta : Subsystem  Description=整车运行状态
      settings: AttributesFormatString=%<Description>
      mask Display: image('整车运行状态.png');
  VentilateMessage : Subsystem  Description=通风报文处理
      settings: AttributesFormatString=%<Description>
      mask Display: image('通风报文处理.png');
  InputSignalBus : Outport
  wires:
  Bus Creator/1 -> InputSignalBus/1
  Rte_SignalBUs/1 -> Bus Selector6/1, Bus Creator/1, Bus Selector4/1, Bus Selector7/1, Bus Selector8/1, Bus Selector/1, Bus Selector9/1, Bus Selector3/1, Bus Selector5/1, Bus Selector2/1, Bus Selector1/1  "Rte_SignalBUs"
  Bus Selector/2 -> RemoteMode/2(HeatAdj_TboxRemoteSts)  "<HeatAdj_TboxRemoteSts>"
  Bus Selector/1 -> RemoteMode/1(HeatAdj_RemoteEnableConfig)  "<HeatAdj_RemoteEnableConfig>"
  Bus Selector/3 -> RemoteMode/3(HeatAdj_RemoteMsgLostFlag)  "<HeatAdj_RemoteMsgLostFlag>"
  Bus Selector1/1 -> EngineRunning/1(HeatAdj_PlatformEngineEnableConfig)  "<HeatAdj_PlatformEngineEnableConfig>"
  Bus Selector1/2 -> EngineRunning/2(HeatAdj_P20_PHEV_EngineCfg)  "<HeatAdj_P20_PHEV_EngineCfg>"
  Bus Selector1/3 -> EngineRunning/3(HeatAdj_ECMD_EngineStatus)  "<HeatAdj_ECMD_EngineStatus>"
  Bus Selector2/1 -> VentilateMessage/1(HeatAdj_CarType)  "<HeatAdj_CarType>"
  Bus Selector2/2 -> VentilateMessage/2(HeatAdj_Driver_HMI_VentilateMsg)  "<HeatAdj_Driver_HMI_VentilateMsg>"
  Bus Selector2/3 -> VentilateMessage/3(HeatAdj_Driver_Tbox_VentilateMsg)  "<HeatAdj_Driver_Tbox_VentilateMsg>"
  Bus Selector2/4 -> VentilateMessage/4(HeatAdj_Passenger_HMI_VentilateMsg)  "<HeatAdj_Passenger_HMI_VentilateMsg>"
  Bus Selector2/5 -> VentilateMessage/5(HeatAdj_Passenger_Tbox_VentilateMsg)  "<HeatAdj_Passenger_Tbox_VentilateMsg>"
  Bus Selector2/6 -> VentilateMessage/6(HeatAdj_Third_HMI_VentilateMsg)  "<HeatAdj_Third_Tbox_VentilateMsg>"
  Bus Selector2/7 -> VentilateMessage/7(HeatAdj_Third_Tbox_VentilateMsg)  "<HeatAdj_Third_HMI_VentilateMsg>"
  RemoteMode/1(RemoteModeFlag) -> Delay/1, Bus Creator/8
  Delay/1 -> [RemoteModeFlag]
  [RemoteModeFlag] -> VentilateMessage/8(RemoteModeFlag)
  EngineRunning/1("EngineRunningFlag ") -> Bus Creator/9, [EngineRunningFlag]
  VentilateMessage/2(PassengerVentilateValid) -> [PassengerVentilateValid], Bus Creator1/2
  VentilateMessage/3(ThirdVentilateValid) -> [ThirdVentilateValid], Bus Creator1/3
  VentilateMessage/1(DriverVentilateValid) -> [DriverVentilateValid], Bus Creator1/1
  Bus Creator1/1 -> Bus Creator/10  "VentValid"
  Bus Selector3/2 -> EorrorProcess/2(HeatAdj_DriverNTCFaultSts)  "<HeatAdj_DriverNTCFaultSts>"
  Bus Selector3/1 -> EorrorProcess/1(HeatAdj_DriverCmdFaultSts)  "<HeatAdj_DriverCmdFaultSts>"
  Bus Selector3/5 -> EorrorProcess/5(HeatAdj_ThirdCmdFaultSts)  "<HeatAdj_ThirdCmdFaultSts>"
  Bus Selector3/6 -> EorrorProcess/6(HeatAdj_ThirdNTCFaultSts)  "<HeatAdj_ThirdNTCFaultSts>"
  EorrorProcess/1("DriverHeatError ") -> Bus Creator2/1
  EorrorProcess/2("PassengerHeatError ") -> Bus Creator2/2
  EorrorProcess/3("ThirdHeatError ") -> Bus Creator2/3
  Bus Creator2/1 -> Bus Creator/12  "HeatError"
  Bus Selector3/3 -> EorrorProcess/3(HeatAdj_PassengerCmdFaultSts)  "<HeatAdj_PassengerCmdFaultSts>"
  Bus Selector3/4 -> EorrorProcess/4(HeatAdj_PassengerNTCFaultSts)  "<HeatAdj_PassengerNTCFaultSts>"
  MaxTime/1(HeatRunMaxTime) -> Bus Creator/2  "HeatRunMaxTime"
  Bus Selector4/1 -> MaxTime/1(HeatAdj_CarType)  "<HeatAdj_CarType>"
  Bus Selector5/2 -> HeatMessage/2(HeatAdj_DriverTbox_Message)  "<HeatAdj_DriverTbox_Message>"
  Bus Selector5/1 -> HeatMessage/1(HeatAdj_DriverHMI_Message)  "<HeatAdj_DriverHMI_Message>"
  Bus Selector5/3 -> HeatMessage/3(HeatAdj_PassengerHMI_Message)  "<HeatAdj_PassengerHMI_Message>"
  Bus Selector5/4 -> HeatMessage/4(HeatAdj_PassengerTbox_Message)  "<HeatAdj_PassengerTbox_Message>"
  Bus Selector5/5 -> HeatMessage/5(HeatAdj_ThirdHMI_Message)  "<HeatAdj_ThirdHMI_Message>"
  Bus Selector5/6 -> HeatMessage/6(HeatAdj_ThirdTbox_Message)  "<HeatAdj_ThirdTbox_Message>"
  [DriverVentilateValid] -> HeatMessage/8(DriverVentilateValid)
  [PassengerVentilateValid] -> HeatMessage/9(PassengerVentilateValid)
  [ThirdVentilateValid] -> HeatMessage/10(ThirdVentilateValid)
  HeatMessage/3(PassengerHMI_Message) -> Bus Creator3/3
  HeatMessage/2(DriverTbox_Message) -> Bus Creator3/2
  HeatMessage/4(PassengerTbox_Message) -> Bus Creator3/4
  HeatMessage/1(DriverHMI_Message) -> Bus Creator3/1
  HeatMessage/5(ThirdHMI_Message) -> Bus Creator3/5
  HeatMessage/6(ThirdTbox_Message) -> Bus Creator3/6
  Bus Creator3/1 -> Bus Creator/11  "HeatMessage"
  Bus Selector6/1 -> VehRunSta/1(HeatAdj_PlatformVehicleEnableConfig)  "<HeatAdj_PlatformVehicleEnableConfig>"
  Bus Selector6/2 -> VehRunSta/2(HeatAdj_P20_PHEV_EngineCfg)  "<HeatAdj_P20_PHEV_EngineCfg>"
  Bus Selector6/3 -> VehRunSta/3(HeatAdj_VCU_VehRunSta)  "<HeatAdj_VCU_VehRunSta>"
  VehRunSta/1("VehicleRunFlag ") -> [VehicleRunFlag], Bus Creator/7
  Bus Selector5/7 -> HeatMessage/7(HeatAdj_CarType)  "<HeatAdj_CarType>"
  Bus Selector7/1 -> HeatAndVentlateConfig/1(HeatAdj_CarType)  "<HeatAdj_CarType>"
  Bus Selector7/2 -> HeatAndVentlateConfig/2(HeatAdj_MemIndexDrHeatConfig)  "<HeatAdj_MemIndexDrHeatConfig>"
  Bus Selector7/3 -> HeatAndVentlateConfig/3(HeatAdj_MemIndexPaHeatConfig)  "<HeatAdj_MemIndexPaHeatConfig>"
  Bus Selector7/4 -> HeatAndVentlateConfig/4(HeatAdj_MemIndexThirdHeatConfig)  "<HeatAdj_MemIndexThirdHeatConfig>"
  Bus Selector7/5 -> HeatAndVentlateConfig/5(HeatAdj_MemDiagDrHeatConfig)  "<HeatAdj_MemDiagDrHeatConfig>"
  Bus Selector7/6 -> HeatAndVentlateConfig/6(HeatAdj_MemDiagPaHeatConfig)  "<HeatAdj_MemDiagPaHeatConfig>"
  Bus Selector7/7 -> HeatAndVentlateConfig/7(HeatAdj_MemDiagThirdHeatConfig)  "<HeatAdj_MemDiagThirdHeatConfig>"
  Bus Selector7/8 -> HeatAndVentlateConfig/8(HeatAdj_DriverVentEnableConfig)  "<HeatAdj_DriverVentEnableConfig>"
  Bus Selector7/9 -> HeatAndVentlateConfig/9(HeatAdj_PassengerVentEnableConfig)  "<HeatAdj_PassengerVentEnableConfig>"
  Bus Selector7/10 -> HeatAndVentlateConfig/10(HeatAdj_ThirdVentEnableConfig)  "<HeatAdj_ThirdVentEnableConfig>"
  HeatAndVentlateConfig/1(HeatConfig) -> Bus Creator/4  "HeatConfig"
  HeatAndVentlateConfig/2(VentConfig) -> [VentConfig], Bus Creator/5  "VentConfig"
  Bus Selector1/4 -> EngineRunning/4(HeatAdj_CarType)  "<HeatAdj_CarType>"
  Bus Selector6/4 -> VehRunSta/4(HeatAdj_CarType)  "<HeatAdj_CarType>"
  Bus Selector8/1 -> DCDC_SwitchSts/1(HeatAdj_CarType)  "<HeatAdj_CarType>"
  Bus Selector8/2 -> DCDC_SwitchSts/2(HeatAdj_DCDCSwitchSts)  "<HeatAdj_DCDCSwitchSts>"
  DCDC_SwitchSts/1(DCDC_SwitchEnable) -> [DCDC_SwitchEnable], Bus Creator/6  "DCDC_SwitchEnable"
  Bus Selector9/1 -> CommonPreconditionDeal/1(HeatAdj_PowerMode)  "<HeatAdj_PowerMode>"
  [DCDC_SwitchEnable] -> CommonPreconditionDeal/3(DCDC_SwitchEnable)
  [EngineRunningFlag] -> CommonPreconditionDeal/4(EngineRunningFlag)
  [VehicleRunFlag] -> CommonPreconditionDeal/5(VehicleRunFlag)
  CommonPreconditionDeal/1("ComPCSatisfiedFlag ") -> Bus Creator/13  "ComPCSatisfiedFlag"
  Bus Selector3/7 -> EorrorProcess/7(HeatAdj_DriverCmdFaultSts4DTC)  "<HeatAdj_DriverCmdFaultSts4DTC>"
  Bus Selector3/8 -> EorrorProcess/8(HeatAdj_PassengerCmdFaultSts4DTC)  "<HeatAdj_PassengerCmdFaultSts4DTC>"
  Bus Selector3/9 -> EorrorProcess/9(HeatAdj_ThirdCmdFaultSts4DTC)  "<HeatAdj_ThirdCmdFaultSts4DTC>"
  EorrorProcess/4(DriverHeatErrorDtc) -> Bus Creator2/4
  EorrorProcess/5(PassengerHeatErrorDtc) -> Bus Creator2/5
  EorrorProcess/6(ThirdHeatErrorDtc) -> Bus Creator2/6
  HeatMessage/7(Driver_MixConflicFlg) -> Bus Creator3/7
  HeatMessage/8(Passenger_MixConflicFlg) -> Bus Creator3/8
  HeatMessage/9(Third_MixConflicFlg) -> Bus Creator3/9
  Bus Selector9/2 -> CommonPreconditionDeal/2(HeatAdj_VoltMode)  "<HeatAdj_VoltMode>"
  Bus Selector4/2 -> MaxTime/2(HeatAdj_ThirdDiagMaxTime)  "<HeatAdj_ThirdDiagMaxTime>"
  MaxTime/2(SwHeatRunMaxTime) -> Bus Creator/3  "SwHeatRunMaxTime"
  Bus Selector7/11 -> HeatAndVentlateConfig/11(HeatAdj_MemDiagDrHeatFlg)  "<HeatAdj_MemDiagDrHeatFlg>"
  Bus Selector7/12 -> HeatAndVentlateConfig/12(HeatAdj_MemDiagPaHeatFlg)  "<HeatAdj_MemDiagPaHeatFlg>"
  [VentConfig] -> VentilateMessage/9(VentConfig)
  Bus Selector7/13 -> HeatAndVentlateConfig/13(HeatAdj_DrVentFlg)  "<HeatAdj_DrVentFlg>"
  Bus Selector7/14 -> HeatAndVentlateConfig/14(HeatAdj_PaVentFlg)  "<HeatAdj_PaVentFlg>"
